simulink model "BS_sim"  (R2019b)
settings: Solver=VariableStepAuto  StartTime=0.0  StopTime=50  RelTol=1e-3
libraries: simulink x1
settings Model: Creator=14351  LastModifiedBy=14351

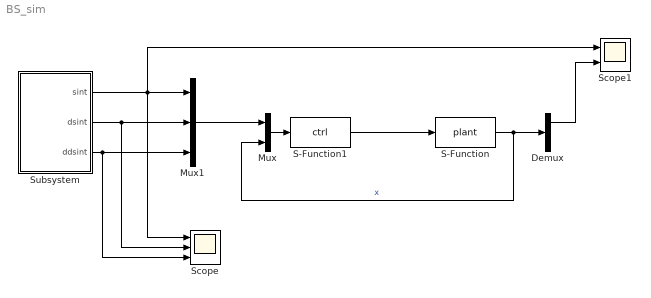
== system BS_sim ==
  Demux : Demux  Outputs=2
  Mux : Mux  Inputs=2
  Mux1 : Mux  Inputs=3
  S-Function : S-Function  FunctionName=plant  Parameters=Pa  SFunctionDeploymentMode=off  EnableBusSupport=off
  S-Function1 : S-Function  FunctionName=ctrl  Parameters=Pa  SFunctionDeploymentMode=off  EnableBusSupport=off
  Scope : Scope  NumInputPorts=3
  Scope1 : Scope  NumInputPorts=2
  Subsystem : Subsystem
  wires:
  S-Function/1 -> Mux/2, Demux/1  "x"
  S-Function1/1 -> S-Function/1
  Mux/1 -> S-Function1/1
  Subsystem/1(sint) -> Scope1/1, Mux1/1, Scope/1
  Subsystem/2(dsint) -> Mux1/2, Scope/2
  Subsystem/3(ddsint) -> Scope/3, Mux1/3
  Demux/1 -> Scope1/2
  Mux1/1 -> Mux/1

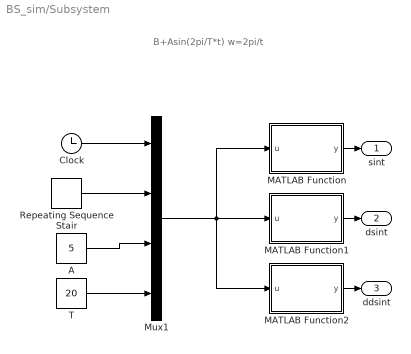
== system BS_sim/Subsystem ==
  note: B+Asin(2pi/T*t)
      | w=2pi/t
  A : Constant  Value=5
  Clock : Clock
      settings: Decimation=50
  MATLAB Function : MATLAB Function  TreatAsAtomicUnit=on
  MATLAB Function1 : MATLAB Function  TreatAsAtomicUnit=on
  MATLAB Function2 : MATLAB Function  TreatAsAtomicUnit=on
  Mux1 : Mux
  Repeating Sequence Stair : simulink/Sources/Repeating Sequence Stair  OutValues=0  tsamp=20  OutMin=[]  OutMax=[]  OutDataTypeStr=double  OutputDataTypeScalingMode=double  OutDataType=fixdt(0,8)  ConRadixGroup=Best Precision: Vector-wise  OutScaling=2^-12
  T : Constant  Value=20
  sint : Outport
  dsint : Outport  Port=2
  ddsint : Outport  Port=3
  wires:
  T/1 -> Mux1/4
  Repeating Sequence Stair/1 -> Mux1/2
  Mux1/1 -> MATLAB Function2/1(u), MATLAB Function1/1(u), MATLAB Function/1(u)
  Clock/1 -> Mux1/1
  MATLAB Function2/1(y) -> ddsint/1
  MATLAB Function/1(y) -> sint/1
  MATLAB Function1/1(y) -> dsint/1
  A/1 -> Mux1/3

== matlab function BS_sim/Subsystem/MATLAB Function1 ==
  data: u input; y output
function y = fcn(u)

y = 2*pi/u(4)*u(3)*cos(2*pi/u(4)*u(1));

== matlab function BS_sim/Subsystem/MATLAB Function ==
  data: u input; y output
function y = fcn(u)

y = u(2)+u(3)*sin(2*pi/u(4)*u(1));

== matlab function BS_sim/Subsystem/MATLAB Function2 ==
  data: u input; y output
function y = fcn(u)

y = -4*pi*pi/u(4)/u(4)*u(3)*sin(2*pi/u(4)*u(1));;
